simulink model "TestYaw"  (R2016a)
settings: Solver=FixedStepAuto  StartTime=0.0  StopTime=inf  RelTol=1e-3
libraries: SimuCopterToolbox x2
settings Model: SimulationMode=external  Creator=IceDragon  LastModifiedBy=IceDragon
settings SolverCC: PositivePriorityOrder=on
settings OptimizationCC: OptimizeModelRefInitCode=on  LifeSpan=1  MaxStackSize=64
settings HardwareCC: ProdBitPerPointer=32  ProdLargestAtomicInteger=Long  ProdLargestAtomicFloat=Double  ProdWordSize=32  ProdHWDeviceType=ARM Compatible->ARM Cortex
settings RTWCC: SystemTargetFile=ert.tlc  HardwareBoard=Raspberry Pi  TemplateMakefile=ert_default_tmf  CustomInclude=bridge simucopter  CustomSource=simucopter-agent.cpp BridgeClient.cpp ZmqBridgeMessageSerializer.cpp AbstractBridgeCommandHandler.cpp BridgeMessage.cpp  CustomDefine=SIMULINK_AGENT  CustomInitializer=simucopter_init();  CustomTerminator=simucopter_stop();  Toolchain=GNU GCC Raspberry Pi  BuildConfiguration=Specify  TargetLang=C++
settings CodeAppCC: ForceParamTrailComments=on  OperatorAnnotations=on  SimulinkDataObjDesc=on  SFDataObjDesc=on  MATLABFcnDesc=on  MangleLength=10  InsertBlockDesc=on  MATLABSourceComments=on
settings ERTTargetCC: SupportVariableSizeSignals=on  ExtModeMexArgs='10.66.66.254' 0 17725  RootIOFormat=Structure reference  IndentSize=4

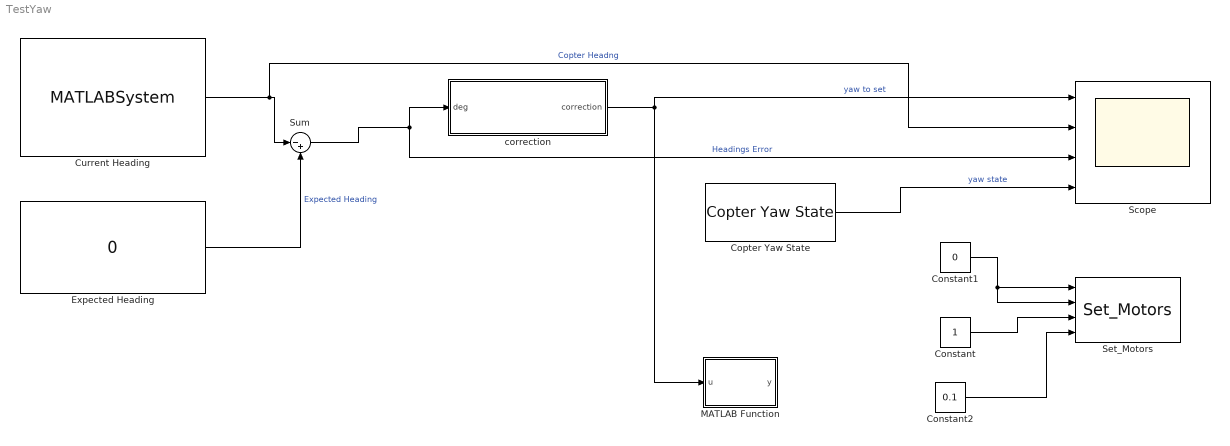
== system TestYaw ==
  Constant : Constant
  Constant1 : Constant  Value=0
  Constant2 : Constant  Value=0.1
  Copter Yaw State : SimuCopterToolbox/Copter Yaw State  SimulateUsing=Code generation
  Current Heading : MATLABSystem  System=copter_heading  SimulateUsing=Code generation
      mask Type: copter_heading
      mask Display:
      | disp('copter_heading');
      | port_label('output',1,'degrees');
  Expected Heading : Constant  Value=0
  MATLAB Function : MATLAB Function  TreatAsAtomicUnit=on
  Scope : Scope  NumInputPorts=4
  Set_Motors : SimuCopterToolbox/Set_Motors  SimulateUsing=Code generation
  Sum : Sum  Inputs=|-+
  correction : MATLAB Function  TreatAsAtomicUnit=on
  wires:
  Current Heading/1 -> Scope/2, Sum/1  "Copter Headng"
  Copter Yaw State/1 -> Scope/4  "yaw state"
  Sum/1 -> Scope/3, correction/1(deg)  "Headings Error"
  correction/1(correction) -> MATLAB Function/1(u), Scope/1  "yaw to set"
  Expected Heading/1 -> Sum/2  "Expected Heading"
  Constant1/1 -> Set_Motors/1, Set_Motors/2
  Constant/1 -> Set_Motors/3
  Constant2/1 -> Set_Motors/4

== matlab function TestYaw/MATLAB Function ==
  data: u input; y output
function y = fcn(u)
%#codegen
if (u == 0)
    y = 0;
else
    y = 0.1;
end
end

== matlab function TestYaw/correction ==
  data: deg input; correction output
function correction = fcn(deg)

    if(deg < -20)
       correction = -1; 
    else if (deg > 20)
       correction = 1;
    else
       correction = 0;
    end
    
end
